simulink model "single_in_out_1t"  (R2021b)
settings: Solver=VariableStepAuto  StartTime=0.0  StopTime=10.0  RelTol=1e-3
settings Model: Creator=den  LastModifiedBy=den

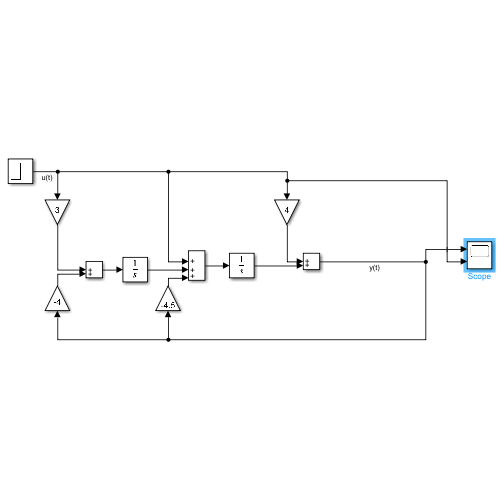
[thumbnail: Simulink's stored preview of the top-level diagram]
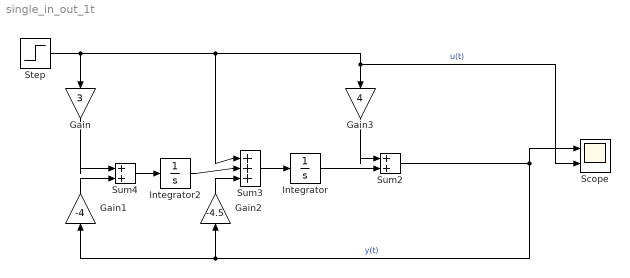
== system single_in_out_1t ==
  Gain : Gain  Gain=3
  Gain1 : Gain  Gain=-4
  Gain2 : Gain  Gain=-4.5
  Gain3 : Gain  Gain=4
  Integrator : Integrator
  Integrator2 : Integrator
  Scope : Scope  NumInputPorts=2
  Step : Step  Time=0  SampleTime=0
  Sum2 : Sum  Inputs=|++
  Sum3 : Sum  Inputs=|+++
  Sum4 : Sum  Inputs=|++
  wires:
  Gain3/1 -> Sum2/1
  Sum2/1 -> Scope/1, Gain1/1, Gain2/1  "y(t)"
  Sum3/1 -> Integrator/1
  Integrator/1 -> Sum2/2
  Gain/1 -> Sum4/1
  Gain1/1 -> Sum4/2
  Sum4/1 -> Integrator2/1
  Gain2/1 -> Sum3/3
  Integrator2/1 -> Sum3/2
  Step/1 -> Scope/2, Gain3/1, Sum3/1, Gain/1  "u(t)"
